simulink model "ReplayAltFilter_oldAtlFilter"  (Simulink 7.8)
settings: Solver=FixedStepDiscrete  StartTime=0.0  StopTime=time(end)  FixedStep=.01  RelTol=1e-3
values from neighbouring files (symbols this model uses):
  apSampleTime = 0.01    [Load_Replay.m]    (also in loadReplayMay2013.m; loadTuneRollReplay_May2013.m; replayFlight.m)
  baroCutoff = 0.2/(2*pi)    (= 0.0318309886184)    [replayFlight.m]
  GS_location = [180 36.9898376464844 -122.051963806152]    [Load_Replay.m]    (also in loadReplayMay2013.m; loadTuneRollReplay_May2013.m; replayFlight.m = [0 36.9898376464844 -122.051963806152])
  ISA_rho0 = 1.225    [replayFlight.m]
  TData = 0.01    [Load_Replay.m]    (also in loadReplayMay2013.m; loadTuneRollReplay_May2013.m)
  Ts = apSampleTime    (= 0.01)    [Load_Replay.m]    (also in loadReplayMay2013.m; loadTuneRollReplay_May2013.m)
  zCutoff = .2    (= 0.2)    [replayFlight.m]
undefined symbols (not defined in the file or in its folder): gaind, polesd, zerosd
libraries: simulink x3
settings Model: Creator=Administrator  LastModifiedBy=Ren
settings OptimizationCC: InitFltsAndDblsToZero=on
settings DebuggingCC: SaveWithParameterizedLinksMsg=none  FcnCallInpInsideContextMsg=Use local settings  StrictBusMsg=Warning
settings SFSimCC: SimParseCustomCode=off
settings GRTTargetCC: TargetFcnLib=ansi_tfl_tmw.mat

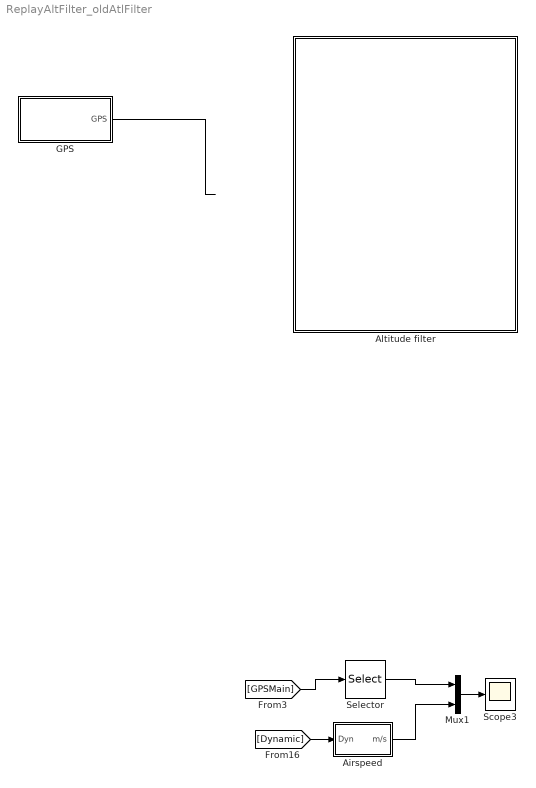
== system ReplayAltFilter_oldAtlFilter ==
  Airspeed : Subsystem
  Altitude filter : Subsystem
  GPS : Subsystem
  Mux1 : Mux  Inputs=2
  Scope3 : Scope
      settings: YMin=0  YMax=22.5  SaveName=ScopeData7
  Selector : Selector  InputPortWidth=5  IndexOptions=Index vector (dialog)  Indices=5  OutputSizes=1
  wires:
  GPS/1(GPS) -> ?
  ? -> ?
  [Dynamic] -> Airspeed/1(Dyn)
  [GPSMain] -> Selector/1
  Selector/1 -> Mux1/1
  Airspeed/1(m/s) -> Mux1/2
  Mux1/1 -> Scope3/1

== system ReplayAltFilter_oldAtlFilter/Airspeed ==
  Dyn : Inport
  Gain : Gain  Gain=2/ISA_rho0
  Math Function : Math  Operator=sqrt  SaturateOnIntegerOverflow=on
  "[0.001  2000]" : Saturate  UpperLimit=2000  LowerLimit=0.001
  m/s : Outport
  wires:
  "[0.001  2000]"/1 -> Math Function/1
  Math Function/1 -> m/s/1
  Dyn/1 -> Gain/1
  Gain/1 -> "[0.001  2000]"/1

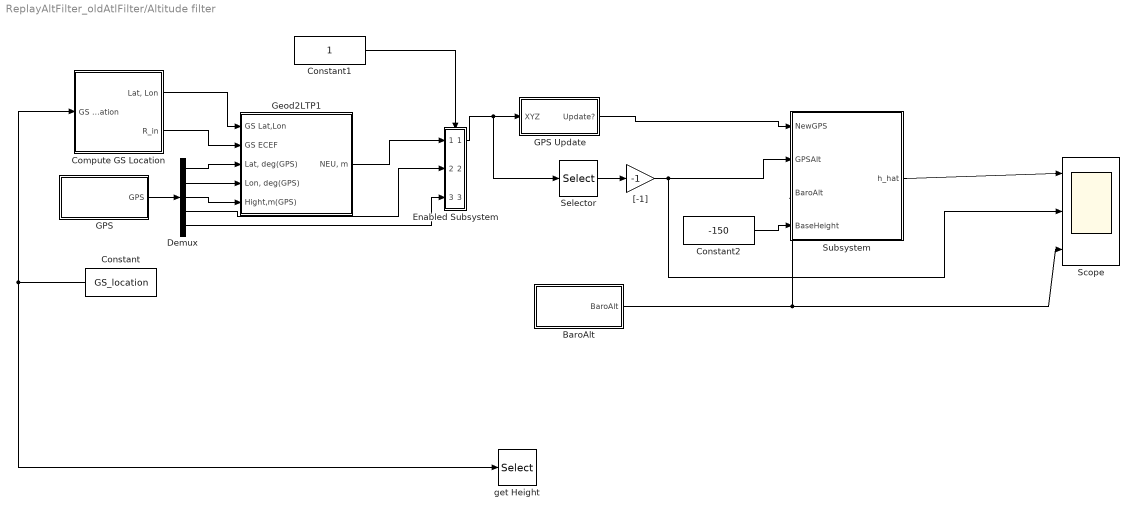
== system ReplayAltFilter_oldAtlFilter/Altitude filter ==
  BaroAlt : Subsystem
  Compute GS Location : Subsystem
  Constant : Constant  Value=GS_location  OutDataTypeStr=single
  Constant1 : Constant  OutDataTypeStr=single
  Constant2 : Constant  Value=-150  OutDataTypeStr=single
  Demux : Demux  Outputs=5
  Enabled Subsystem : Subsystem  TreatAsAtomicUnit=on
  GPS : Subsystem
  GPS Update : Subsystem  mask{T=0.01}
      mask prompts: T "Sample Time"
  Geod2LTP1 : Subsystem
      mask Description:
      | This block provides transformation of the Geodetic coordinates
      | to the LTP coorinate system. The block uses two consecutive transformations
      | (Geodetic -> ECEF ->LTP).
      | Geodetic coordinates of the LTP origin should also be predetermined.
      mask Help: Oops!
      mask Display: plot(0,0,100,100,[45,40,35,40,40],[85,95,85,95,40],[85,95,85,95,40],[35,40,45,40,40],[60,40,10,20,10,14],[70,40,10,13,10,20],[56,45],[70,70],[60,60],[50,60],[60,60],[30,40],[50,60],[20,20],[30,40],[20,20],[45,55],[35,25],[75,65],[35,25])
  Scope : Scope  NumInputPorts=3
      settings: YMin=98550~-50~98550  YMax=99200~15~99300
  Selector : Selector  InputPortWidth=3  IndexOptions=Index vector (dialog)  Indices=[3]  OutputSizes=1
  Subsystem : Subsystem
  "[-1]" : Gain  Gain=-1
  get Height : Selector  InputPortWidth=3  IndexOptions=Index vector (dialog)  Indices=[1]  OutputSizes=1
  wires:
  Constant/1 -> Compute GS Location/1(GS Location), get Height/1
  Demux/1 -> Geod2LTP1/3("Lat, deg(GPS)")
  Demux/2 -> Geod2LTP1/4("Lon, deg(GPS)")
  Demux/3 -> Geod2LTP1/5(Hight,m(GPS))
  Compute GS Location/2(R_in) -> Geod2LTP1/2(GS ECEF)
  Compute GS Location/1("Lat, Lon") -> Geod2LTP1/1(GS Lat,Lon)
  GPS Update/1(Update?) -> Subsystem/1(NewGPS)
  Constant1/1 -> Enabled Subsystem/Enable
  Enabled Subsystem/1(Out1) -> GPS Update/1(XYZ), Selector/1
  Geod2LTP1/1("NEU, m") -> Enabled Subsystem/1(In1)
  Demux/4 -> Enabled Subsystem/2(In2)
  Demux/5 -> Enabled Subsystem/3(In3)
  Subsystem/1(h_hat) -> Scope/1
  Constant2/1 -> Subsystem/4(BaseHeight)
  BaroAlt/1(BaroAlt) -> Subsystem/3(BaroAlt), Scope/3
  "[-1]"/1 -> Subsystem/2(GPSAlt), Scope/2
  Selector/1 -> "[-1]"/1
  GPS/1(GPS) -> Demux/1

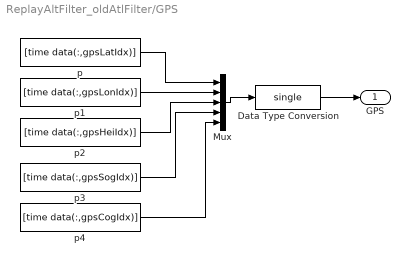
== system ReplayAltFilter_oldAtlFilter/GPS ==
  Data Type Conversion : DataTypeConversion  OutDataTypeStr=single
  Mux : Mux  Inputs=5
  p : FromWorkspace  VariableName=[time data(:,gpsLatIdx)]  SampleTime=TData  OutputAfterFinalValue=Setting to zero
  p1 : FromWorkspace  VariableName=[time data(:,gpsLonIdx)]  SampleTime=TData  OutputAfterFinalValue=Setting to zero
  p2 : FromWorkspace  VariableName=[time data(:,gpsHeiIdx)]  SampleTime=TData  OutputAfterFinalValue=Setting to zero
  p3 : FromWorkspace  VariableName=[time data(:,gpsSogIdx)]  SampleTime=Ts  OutputAfterFinalValue=Setting to zero
  p4 : FromWorkspace  VariableName=[time data(:,gpsCogIdx)]  SampleTime=TData  OutputAfterFinalValue=Setting to zero
  GPS : Outport
  wires:
  p/1 -> Mux/1
  p1/1 -> Mux/2
  p2/1 -> Mux/3
  Mux/1 -> Data Type Conversion/1
  p3/1 -> Mux/4
  p4/1 -> Mux/5
  Data Type Conversion/1 -> GPS/1

== system ReplayAltFilter_oldAtlFilter/Altitude filter/BaroAlt ==
  Data Type Conversion : DataTypeConversion  OutDataTypeStr=single
  p1 : FromWorkspace  VariableName=[time data(:,airStaIdx)]  SampleTime=apSampleTime  OutputAfterFinalValue=Setting to zero
  BaroAlt : Outport
  wires:
  Data Type Conversion/1 -> BaroAlt/1
  p1/1 -> Data Type Conversion/1

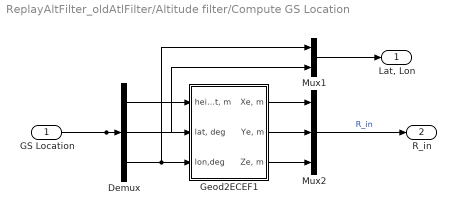
== system ReplayAltFilter_oldAtlFilter/Altitude filter/Compute GS Location ==
  GS Location : Inport
  Demux : Demux  Outputs=3
  Geod2ECEF1 : Subsystem  mask{Re=6378137, Rp=6356752.3142}
      mask prompts: Re "Enter equatorial radius, m"; Rp "Enter polar radius,m"
  Mux1 : Mux  Inputs=2
  Mux2 : Mux  Inputs=3
  "Lat, Lon" : Outport
  R_in : Outport  Port=2
  wires:
  Geod2ECEF1/3("Ze, m ") -> Mux2/3
  Geod2ECEF1/1("Xe, m ") -> Mux2/1
  Geod2ECEF1/2("Ye, m ") -> Mux2/2
  Demux/1 -> Geod2ECEF1/1("height, m")
  Demux/2 -> Mux1/2, Geod2ECEF1/2("lat, deg")
  Demux/3 -> Mux1/1, Geod2ECEF1/3(lon,deg)
  GS Location/1 -> Demux/1
  Mux1/1 -> "Lat, Lon"/1
  Mux2/1 -> R_in/1  "R_in"

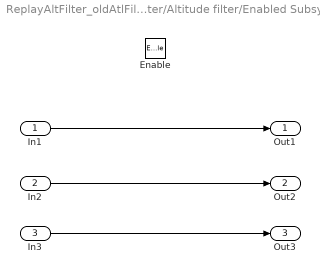
== system ReplayAltFilter_oldAtlFilter/Altitude filter/Enabled Subsystem ==
  In1 : Inport
  In2 : Inport  Port=2
  In3 : Inport  Port=3
  Enable : EnablePort
  Out1 : Outport
  Out2 : Outport  Port=2
  Out3 : Outport  Port=3
  wires:
  In1/1 -> Out1/1
  In2/1 -> Out2/1
  In3/1 -> Out3/1

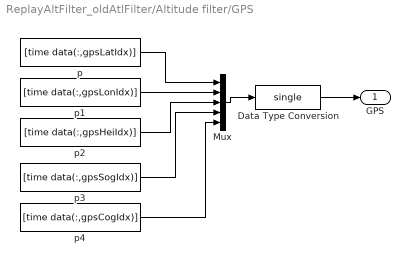
== system ReplayAltFilter_oldAtlFilter/Altitude filter/GPS ==
  Data Type Conversion : DataTypeConversion  OutDataTypeStr=single
  Mux : Mux  Inputs=5
  p : FromWorkspace  VariableName=[time data(:,gpsLatIdx)]  SampleTime=TData  OutputAfterFinalValue=Setting to zero
  p1 : FromWorkspace  VariableName=[time data(:,gpsLonIdx)]  SampleTime=TData  OutputAfterFinalValue=Setting to zero
  p2 : FromWorkspace  VariableName=[time data(:,gpsHeiIdx)]  SampleTime=TData  OutputAfterFinalValue=Setting to zero
  p3 : FromWorkspace  VariableName=[time data(:,gpsSogIdx)]  SampleTime=Ts  OutputAfterFinalValue=Setting to zero
  p4 : FromWorkspace  VariableName=[time data(:,gpsCogIdx)]  SampleTime=TData  OutputAfterFinalValue=Setting to zero
  GPS : Outport
  wires:
  p/1 -> Mux/1
  p1/1 -> Mux/2
  p2/1 -> Mux/3
  Mux/1 -> Data Type Conversion/1
  p3/1 -> Mux/4
  p4/1 -> Mux/5
  Data Type Conversion/1 -> GPS/1

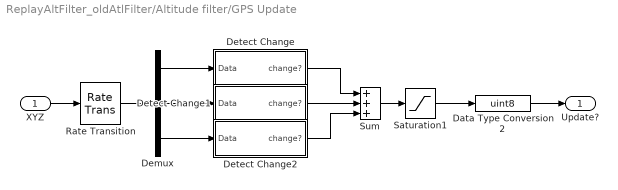
== system ReplayAltFilter_oldAtlFilter/Altitude filter/GPS Update ==
  XYZ : Inport
  Data Type Conversion2 : DataTypeConversion  OutDataTypeStr=uint8
  Demux : Demux  Outputs=3
  Detect Change : Subsystem
  Detect Change1 : Subsystem
  Detect Change2 : Subsystem
  Rate Transition : RateTransition  OutPortSampleTime=T
  Saturation1 : Saturate  UpperLimit=1  LowerLimit=0  SampleTime=T
  Sum : Sum  Inputs=3
  Update? : Outport
  wires:
  Demux/1 -> Detect Change/1(Data)
  Demux/2 -> Detect Change1/1(Data)
  Demux/3 -> Detect Change2/1(Data)
  Detect Change/1(change?) -> Sum/1
  Detect Change1/1(change?) -> Sum/2
  Detect Change2/1(change?) -> Sum/3
  Sum/1 -> Saturation1/1
  XYZ/1 -> Rate Transition/1
  Saturation1/1 -> Data Type Conversion2/1
  Rate Transition/1 -> Demux/1
  Data Type Conversion2/1 -> Update?/1

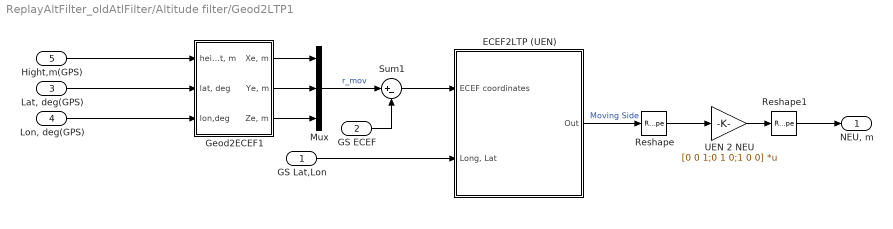
== system ReplayAltFilter_oldAtlFilter/Altitude filter/Geod2LTP1 ==
  GS Lat,Lon : Inport
  GS ECEF : Inport  Port=2
  "Lat, deg(GPS)" : Inport  Port=3
  "Lon, deg(GPS)" : Inport  Port=4
  Hight,m(GPS) : Inport  Port=5
  ECEF2LTP (UEN) : Subsystem
      mask Display: plot(0,0,100,100,[45,40,35,40,40],[85,95,85,95,40],[85,95,85,95,40],[35,40,45,40,40],[60,40,10,20,10,14],[70,40,10,13,10,20],[56,45],[70,70],[60,60],[50,60],[60,60],[30,40],[50,60],[20,20],[30,40],[20,20],[45,55],[35,25],[75,65],[35,25])
  Geod2ECEF1 : Subsystem  mask{Re=6378137, Rp=6356752.3142}
      mask prompts: Re "Enter equatorial radius, m"; Rp "Enter polar radius,m"
  Mux : Mux  Inputs=3
  Reshape : Reshape  OutputDimensionality=Column vector (2-D)
  Reshape1 : Reshape
  Sum1 : Sum  Inputs=|+-  OutDataTypeStr=single  SaturateOnIntegerOverflow=on
  UEN 2 NEU : Gain  Gain=[0 0 1;0 1 0;1 0 0]  Multiplication=Matrix(K*u)  OutDataTypeStr=float('single')  SaturateOnIntegerOverflow=on  ParamDataTypeStr=Inherit: Same as input
  "NEU, m" : Outport
  wires:
  Reshape1/1 -> "NEU, m"/1
  Reshape/1 -> UEN 2 NEU/1
  Sum1/1 -> ECEF2LTP (UEN)/1(ECEF coordinates)
  Mux/1 -> Sum1/1  "r_mov"
  Hight,m(GPS)/1 -> Geod2ECEF1/1("height, m")
  ECEF2LTP (UEN)/1(Out) -> Reshape/1  "Moving Side"
  GS ECEF/1 -> Sum1/2
  GS Lat,Lon/1 -> ECEF2LTP (UEN)/2("Long, Lat")
  "Lon, deg(GPS)"/1 -> Geod2ECEF1/3(lon,deg)
  "Lat, deg(GPS)"/1 -> Geod2ECEF1/2("lat, deg")
  Geod2ECEF1/2("Ye, m ") -> Mux/2
  Geod2ECEF1/1("Xe, m ") -> Mux/1
  Geod2ECEF1/3("Ze, m ") -> Mux/3
  UEN 2 NEU/1 -> Reshape1/1

== system ReplayAltFilter_oldAtlFilter/Altitude filter/Subsystem ==
  NewGPS : Inport
  GPSAlt : Inport  Port=2
  BaroAlt : Inport  Port=3
  BaseHeight : Inport  Port=4
  2 FIlter Blend : Subsystem
  h_hat : Outport
  wires:
  2 FIlter Blend/1(Blend) -> h_hat/1
  BaseHeight/1 -> 2 FIlter Blend/4(baseHeight)
  BaroAlt/1 -> 2 FIlter Blend/2(BaroAlt)
  GPSAlt/1 -> 2 FIlter Blend/1(gps_h)
  NewGPS/1 -> 2 FIlter Blend/3(New GPS)

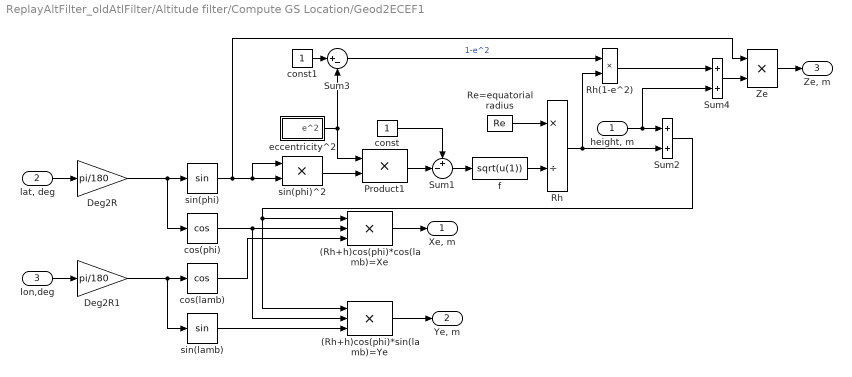
== system ReplayAltFilter_oldAtlFilter/Altitude filter/Compute GS Location/Geod2ECEF1 ==
  "height, m" : Inport
  "lat, deg" : Inport  Port=2
  lon,deg : Inport  Port=3
  (Rh+h)cos(phi)*cos(lamb)=Xe : Product  Inputs=3  OutDataTypeStr=single  SaturateOnIntegerOverflow=on  InputSameDT=on
  (Rh+h)cos(phi)*sin(lamb)=Ye : Product  Inputs=3  OutDataTypeStr=single  SaturateOnIntegerOverflow=on  InputSameDT=on
  Deg2R : Gain  Gain=pi/180  OutDataTypeStr=float('single')  SaturateOnIntegerOverflow=on  ParamDataTypeStr=Inherit: Same as input
  Deg2R1 : Gain  Gain=pi/180  OutDataTypeStr=float('single')  SaturateOnIntegerOverflow=on  ParamDataTypeStr=Inherit: Same as input
  Product1 : Product  SaturateOnIntegerOverflow=on  InputSameDT=on  OutDataTypeStr=Inherit: Same as first input
  Re=equatorial radius : Constant  Value=Re  OutDataTypeStr=single
  Rh : Product  Inputs=*/  OutDataTypeStr=single  SaturateOnIntegerOverflow=on  InputSameDT=on
  Rh(1-e^2) : Product  OutDataTypeStr=single  SaturateOnIntegerOverflow=on  InputSameDT=on
  Sum1 : Sum  Inputs=+-|  SaturateOnIntegerOverflow=on  InputSameDT=on  OutDataTypeStr=Inherit: Same as first input
  Sum2 : Sum  SaturateOnIntegerOverflow=on  InputSameDT=on  OutDataTypeStr=Inherit: Same as first input
      settings: AttributesFormatString=Rh+h
  Sum3 : Sum  Inputs=|+-  SaturateOnIntegerOverflow=on  InputSameDT=on  OutDataTypeStr=Inherit: Same as first input
  Sum4 : Sum  OutDataTypeStr=single  SaturateOnIntegerOverflow=on  InputSameDT=on
      settings: AttributesFormatString=(1-e^2)Rh+h
  Ze : Product  OutDataTypeStr=single  SaturateOnIntegerOverflow=on  InputSameDT=on
  const : Constant  OutDataTypeStr=single
  const1 : Constant  OutDataTypeStr=single
  cos(lamb) : Trigonometry  Operator=cos
  cos(phi) : Trigonometry  Operator=cos
  eccentricity^2 : Subsystem
  f : Fcn  Expr=sqrt(u(1))
  sin(lamb) : Trigonometry
  sin(phi) : Trigonometry
  sin(phi)^2 : Product  SaturateOnIntegerOverflow=on  InputSameDT=on  OutDataTypeStr=Inherit: Same as first input
  "Xe, m " : Outport
  "Ye, m " : Outport  Port=2
  "Ze, m " : Outport  Port=3
  wires:
  (Rh+h)cos(phi)*sin(lamb)=Ye/1 -> "Ye, m "/1
  (Rh+h)cos(phi)*cos(lamb)=Xe/1 -> "Xe, m "/1
  Sum2/1 -> (Rh+h)cos(phi)*cos(lamb)=Xe/1, (Rh+h)cos(phi)*sin(lamb)=Ye/1
  Deg2R1/1 -> sin(lamb)/1, cos(lamb)/1
  Deg2R/1 -> sin(phi)/1, cos(phi)/1
  Ze/1 -> "Ze, m "/1
  sin(lamb)/1 -> (Rh+h)cos(phi)*sin(lamb)=Ye/3
  cos(lamb)/1 -> (Rh+h)cos(phi)*cos(lamb)=Xe/3
  cos(phi)/1 -> (Rh+h)cos(phi)*sin(lamb)=Ye/2, (Rh+h)cos(phi)*cos(lamb)=Xe/2
  lon,deg/1 -> Deg2R1/1
  Sum4/1 -> Ze/2
  Rh(1-e^2)/1 -> Sum4/1
  Sum3/1 -> Rh(1-e^2)/1  "1-e^2"
  const1/1 -> Sum3/1
  sin(phi)^2/1 -> Product1/2
  eccentricity^2/1(e^2) -> Sum3/2, Product1/1
  "height, m"/1 -> Sum2/1, Sum4/2
  const/1 -> Sum1/1
  Sum1/1 -> f/1
  Product1/1 -> Sum1/2
  Rh/1 -> Rh(1-e^2)/2, Sum2/2
  Re=equatorial radius/1 -> Rh/1
  f/1 -> Rh/2
  sin(phi)/1 -> Ze/1, sin(phi)^2/2, sin(phi)^2/1
  "lat, deg"/1 -> Deg2R/1

== system ReplayAltFilter_oldAtlFilter/Altitude filter/GPS Update/Detect Change ==
  Data : Inport
  Abs1 : Abs  SampleTime=T
  Difference1 : simulink/Discrete/Difference  ICPrevInput=0.0  InputProcessing=Inherited  OutMin=[]  OutMax=[]  OutDataType=sfix(16)  OutScaling=2^-10  DoSatur=off
  Saturation1 : Saturate  UpperLimit=1  LowerLimit=0  SampleTime=T
  change? : Outport
  wires:
  Difference1/1 -> Abs1/1
  Abs1/1 -> Saturation1/1
  Data/1 -> Difference1/1
  Saturation1/1 -> change?/1

== system ReplayAltFilter_oldAtlFilter/Altitude filter/GPS Update/Detect Change1 ==
  Data : Inport
  Abs1 : Abs  SampleTime=T
  Difference1 : simulink/Discrete/Difference  ICPrevInput=0.0  InputProcessing=Inherited  OutMin=[]  OutMax=[]  OutDataType=sfix(16)  OutScaling=2^-10  DoSatur=off
  Saturation1 : Saturate  UpperLimit=1  LowerLimit=0  SampleTime=T
  change? : Outport
  wires:
  Saturation1/1 -> change?/1
  Data/1 -> Difference1/1
  Abs1/1 -> Saturation1/1
  Difference1/1 -> Abs1/1

== system ReplayAltFilter_oldAtlFilter/Altitude filter/GPS Update/Detect Change2 ==
  Data : Inport
  Abs1 : Abs  SampleTime=T
  Difference1 : simulink/Discrete/Difference  ICPrevInput=0.0  InputProcessing=Inherited  OutMin=[]  OutMax=[]  OutDataType=sfix(16)  OutScaling=2^-10  DoSatur=off
  Saturation1 : Saturate  UpperLimit=1  LowerLimit=0  SampleTime=T
  change? : Outport
  wires:
  Difference1/1 -> Abs1/1
  Abs1/1 -> Saturation1/1
  Data/1 -> Difference1/1
  Saturation1/1 -> change?/1

== system ReplayAltFilter_oldAtlFilter/Altitude filter/Geod2LTP1/ECEF2LTP (UEN) ==
  ECEF coordinates : Inport
  "Long, Lat" : Inport  Port=2
  Deg2R : Gain  Gain=pi/180  SaturateOnIntegerOverflow=on  OutDataTypeStr=Inherit: Same as input  ParamDataTypeStr=Inherit: Same as input
  Demux3 : Demux  Outputs=2
  From Body to Universal1 : Subsystem
  Product1 : Product  Multiplication=Matrix(*)  SaturateOnIntegerOverflow=on  InputSameDT=on  OutDataTypeStr=Inherit: Same as first input
  Out : Outport
  wires:
  From Body to Universal1/1(DCM) -> Product1/1
  ECEF coordinates/1 -> Product1/2
  Deg2R/1 -> Demux3/1
  Demux3/1 -> From Body to Universal1/1(long)
  Demux3/2 -> From Body to Universal1/2(lat)
  Product1/1 -> Out/1
  "Long, Lat"/1 -> Deg2R/1

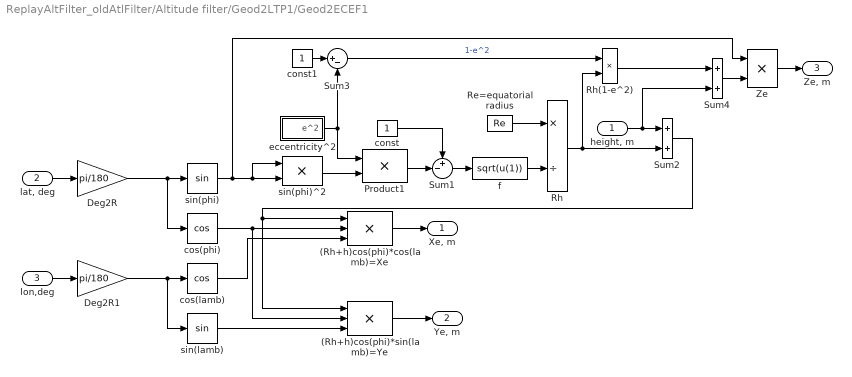
== system ReplayAltFilter_oldAtlFilter/Altitude filter/Geod2LTP1/Geod2ECEF1 ==
  "height, m" : Inport
  "lat, deg" : Inport  Port=2
  lon,deg : Inport  Port=3
  (Rh+h)cos(phi)*cos(lamb)=Xe : Product  Inputs=3  OutDataTypeStr=single  SaturateOnIntegerOverflow=on  InputSameDT=on
  (Rh+h)cos(phi)*sin(lamb)=Ye : Product  Inputs=3  OutDataTypeStr=single  SaturateOnIntegerOverflow=on  InputSameDT=on
  Deg2R : Gain  Gain=pi/180  OutDataTypeStr=float('single')  SaturateOnIntegerOverflow=on  ParamDataTypeStr=Inherit: Same as input
  Deg2R1 : Gain  Gain=pi/180  OutDataTypeStr=float('single')  SaturateOnIntegerOverflow=on  ParamDataTypeStr=Inherit: Same as input
  Product1 : Product  SaturateOnIntegerOverflow=on  InputSameDT=on  OutDataTypeStr=Inherit: Same as first input
  Re=equatorial radius : Constant  Value=Re  OutDataTypeStr=single
  Rh : Product  Inputs=*/  OutDataTypeStr=single  SaturateOnIntegerOverflow=on  InputSameDT=on
  Rh(1-e^2) : Product  OutDataTypeStr=single  SaturateOnIntegerOverflow=on  InputSameDT=on
  Sum1 : Sum  Inputs=+-|  SaturateOnIntegerOverflow=on  InputSameDT=on  OutDataTypeStr=Inherit: Same as first input
  Sum2 : Sum  SaturateOnIntegerOverflow=on  InputSameDT=on  OutDataTypeStr=Inherit: Same as first input
      settings: AttributesFormatString=Rh+h
  Sum3 : Sum  Inputs=|+-  SaturateOnIntegerOverflow=on  InputSameDT=on  OutDataTypeStr=Inherit: Same as first input
  Sum4 : Sum  OutDataTypeStr=single  SaturateOnIntegerOverflow=on  InputSameDT=on
      settings: AttributesFormatString=(1-e^2)Rh+h
  Ze : Product  OutDataTypeStr=single  SaturateOnIntegerOverflow=on  InputSameDT=on
  const : Constant  OutDataTypeStr=single
  const1 : Constant  OutDataTypeStr=single
  cos(lamb) : Trigonometry  Operator=cos
  cos(phi) : Trigonometry  Operator=cos
  eccentricity^2 : Subsystem
  f : Fcn  Expr=sqrt(u(1))
  sin(lamb) : Trigonometry
  sin(phi) : Trigonometry
  sin(phi)^2 : Product  SaturateOnIntegerOverflow=on  InputSameDT=on  OutDataTypeStr=Inherit: Same as first input
  "Xe, m " : Outport
  "Ye, m " : Outport  Port=2
  "Ze, m " : Outport  Port=3
  wires:
  (Rh+h)cos(phi)*sin(lamb)=Ye/1 -> "Ye, m "/1
  (Rh+h)cos(phi)*cos(lamb)=Xe/1 -> "Xe, m "/1
  Sum2/1 -> (Rh+h)cos(phi)*cos(lamb)=Xe/1, (Rh+h)cos(phi)*sin(lamb)=Ye/1
  Deg2R1/1 -> sin(lamb)/1, cos(lamb)/1
  Deg2R/1 -> sin(phi)/1, cos(phi)/1
  Ze/1 -> "Ze, m "/1
  sin(lamb)/1 -> (Rh+h)cos(phi)*sin(lamb)=Ye/3
  cos(lamb)/1 -> (Rh+h)cos(phi)*cos(lamb)=Xe/3
  cos(phi)/1 -> (Rh+h)cos(phi)*sin(lamb)=Ye/2, (Rh+h)cos(phi)*cos(lamb)=Xe/2
  lon,deg/1 -> Deg2R1/1
  Sum4/1 -> Ze/2
  Rh(1-e^2)/1 -> Sum4/1
  Sum3/1 -> Rh(1-e^2)/1  "1-e^2"
  const1/1 -> Sum3/1
  sin(phi)^2/1 -> Product1/2
  eccentricity^2/1(e^2) -> Sum3/2, Product1/1
  "height, m"/1 -> Sum2/1, Sum4/2
  const/1 -> Sum1/1
  Sum1/1 -> f/1
  Product1/1 -> Sum1/2
  Rh/1 -> Rh(1-e^2)/2, Sum2/2
  Re=equatorial radius/1 -> Rh/1
  f/1 -> Rh/2
  sin(phi)/1 -> Ze/1, sin(phi)^2/2, sin(phi)^2/1
  "lat, deg"/1 -> Deg2R/1

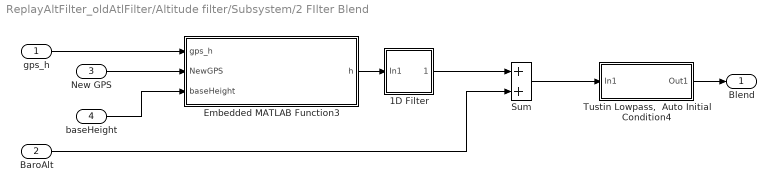
== system ReplayAltFilter_oldAtlFilter/Altitude filter/Subsystem/2 FIlter Blend ==
  gps_h : Inport
  BaroAlt : Inport  Port=2
  New GPS : Inport  Port=3
  baseHeight : Inport  Port=4
  1D Filter : Subsystem  AncestorBlock=SLUGS_Library/Singnal Routing & Conditioning/3D Filter  RTWFcnName=TustinFilter3D  mask{zval=[0], pval=-zCutoff, kval=1, TSample=apSampleTime}
      mask prompts: zval "Zeros"; pval "Poles"; kval "Gains"; TSample "Sample Time"
      settings: RTWFcnNameOpts=User specified  RTWFileNameOpts=Use function name
      mask Display:
      | droots(zval,pval,kval)
      | port_label('input',1,'1D')
  Embedded MATLAB Function3 : MATLAB Function  TreatAsAtomicUnit=on
  Sum : Sum  OutDataTypeStr=single
  "Tustin Lowpass,  Auto Initial Condition4" : Subsystem  mask(Tustin1stOrderLowpassAutoInitialCondition){f=baroCutoff, T=apSampleTime}
      mask prompts: f "Lowpass Frequency"; T "Sample Time"
      mask help: Takes a 3db rolloff frequency (in Hz, NOT radians/s) and a sample time. Performs a symbolic Tustin conversion and implements in a discrete filter. The initial output of the filter is set by the first sample.
      mask Help: Enter the desired 3db rolloff frequency in Hz and the sample time. Initial conditions are sampled automatically.
      mask Display: fprintf('%.2f Hz lowpass',f)
  Blend : Outport
  wires:
  BaroAlt/1 -> Sum/2
  1D Filter/1(Out1) -> Sum/1
  Sum/1 -> "Tustin Lowpass,  Auto Initial Condition4"/1(In1)
  New GPS/1 -> Embedded MATLAB Function3/2(NewGPS)
  gps_h/1 -> Embedded MATLAB Function3/1(gps_h)
  Embedded MATLAB Function3/1(h) -> 1D Filter/1(In1)
  baseHeight/1 -> Embedded MATLAB Function3/3(baseHeight)
  "Tustin Lowpass,  Auto Initial Condition4"/1(Out1) -> Blend/1

== system ReplayAltFilter_oldAtlFilter/Altitude filter/Compute GS Location/Geod2ECEF1/eccentricity^2 ==
  " " : Product  OutDataTypeStr=single  SaturateOnIntegerOverflow=on  InputSameDT=on
  Re=equatorial radius1 : Constant  Value=Re  OutDataTypeStr=single
  Rp=polar radius : Constant  Value=Rp  OutDataTypeStr=single
  Sum5 : Sum  Inputs=|+-  SaturateOnIntegerOverflow=on  InputSameDT=on  OutDataTypeStr=Inherit: Same as first input
  const2 : Constant  OutDataTypeStr=single
  e^1 : Product  Inputs=*/  OutDataTypeStr=single  SaturateOnIntegerOverflow=on  InputSameDT=on
  e^2 : Outport
  wires:
  Sum5/1 -> e^2/1
  " "/1 -> Sum5/2
  e^1/1 -> " "/1, " "/2
  const2/1 -> Sum5/1
  Rp=polar radius/1 -> e^1/1
  Re=equatorial radius1/1 -> e^1/2

== system ReplayAltFilter_oldAtlFilter/Altitude filter/Geod2LTP1/ECEF2LTP (UEN)/From Body to Universal1 ==
  long : Inport
  lat : Inport  Port=2
  Mux : Mux  Inputs=2
  Reshape 9x1->3x1 : Reshape  OutputDimensionality=Customize  OutputDimensions=[3,3]
  Rotation Matrix from Long//Lat : Subsystem
      mask Type: Vector Transformation
      mask Description: Vector Transformation
      mask Display: disp('axis')
  DCM : Outport
  wires:
  Reshape 9x1->3x1/1 -> DCM/1
  Rotation Matrix from Long//Lat/1(DCM) -> Reshape 9x1->3x1/1
  Mux/1 -> Rotation Matrix from Long//Lat/1(long lat)
  long/1 -> Mux/1
  lat/1 -> Mux/2

== system ReplayAltFilter_oldAtlFilter/Altitude filter/Geod2LTP1/Geod2ECEF1/eccentricity^2 ==
  " " : Product  OutDataTypeStr=single  SaturateOnIntegerOverflow=on  InputSameDT=on
  Re=equatorial radius1 : Constant  Value=Re  OutDataTypeStr=single
  Rp=polar radius : Constant  Value=Rp  OutDataTypeStr=single
  Sum5 : Sum  Inputs=|+-  SaturateOnIntegerOverflow=on  InputSameDT=on  OutDataTypeStr=Inherit: Same as first input
  const2 : Constant  OutDataTypeStr=single
  e^1 : Product  Inputs=*/  OutDataTypeStr=single  SaturateOnIntegerOverflow=on  InputSameDT=on
  e^2 : Outport
  wires:
  Sum5/1 -> e^2/1
  " "/1 -> Sum5/2
  e^1/1 -> " "/1, " "/2
  const2/1 -> Sum5/1
  Rp=polar radius/1 -> e^1/1
  Re=equatorial radius1/1 -> e^1/2

== system ReplayAltFilter_oldAtlFilter/Altitude filter/Subsystem/2 FIlter Blend/1D Filter ==
  In1 : Inport
  Data Type Conversion1 : DataTypeConversion  OutDataTypeStr=single
  Data Type Conversion2 : DataTypeConversion  OutDataTypeStr=double
  Filter2 : Subsystem  mask(DiscretizedZeroPole){Zeros=zval, Poles=pval, Gain=kval, AbsTol=auto, SampleTime=TSample, method=tustin, Wc=1}
      mask prompts: Zeros "Zeros (enter in s-main:)"; Poles "Poles (enter in s-domain:)"; Gain "Gain (enter in s-domain:)"; AbsTol "Absolute tolerance:"; SampleTime "Sample time:"; Wc "Critical Frequency (Hz):"
      mask help: Continuous mask uses c2d to transform parameters onto the Discrete Zero-Pole block inside.
      mask init:
      | st=SampleTime;
      | if length(st)>1
      |     st=SampleTime(1);
      | end
      | if(st>0)
      |     [zerosd,polesd,gaind] = sldiscutil('disczpk', {st,method,Wc,Zeros,Poles,Gain});
      | end	
      | s = get_param(gcb,'maskvalues');
      | zeross = s{1};
      | poless = s{2};
      | gainss = s{3};
      | %zerosc = eval(zeross);
      | %polesc = eval(poless);
      | %gainsc = eval(gainss);
      | sldiscutil('initzpkmask', st);
      | if(st==0)
      | set_param([gcb '/Zero Pole'], 'AbsoluteTolerance', AbsTol);
      | end
      mask StyleString: edit,edit,edit,edit,edit,popup(zoh|foh|tustin|prewarp|matched),edit
      mask CallbackString: |||||hidecrit|
      mask Display:
      | droots(zeross,poless,gainss)
      | text( 0.5, 1.0, method, 'verticalAlignment','top')
  Out1 : Outport
  wires:
  Data Type Conversion1/1 -> Out1/1
  Data Type Conversion2/1 -> Filter2/1(In1)
  In1/1 -> Data Type Conversion2/1
  Filter2/1(Out1) -> Data Type Conversion1/1

== system ReplayAltFilter_oldAtlFilter/Altitude filter/Subsystem/2 FIlter Blend/Tustin Lowpass,  Auto Initial Condition4 ==
  In1 : Inport
  Constant : Constant  Value=T
  Constant1 : Constant  Value=f
  Embedded MATLAB Function : MATLAB Function  TreatAsAtomicUnit=on
  Out1 : Outport
  wires:
  Constant/1 -> Embedded MATLAB Function/2(T)
  Constant1/1 -> Embedded MATLAB Function/3(f)
  Embedded MATLAB Function/1(y) -> Out1/1
  In1/1 -> Embedded MATLAB Function/1(u)

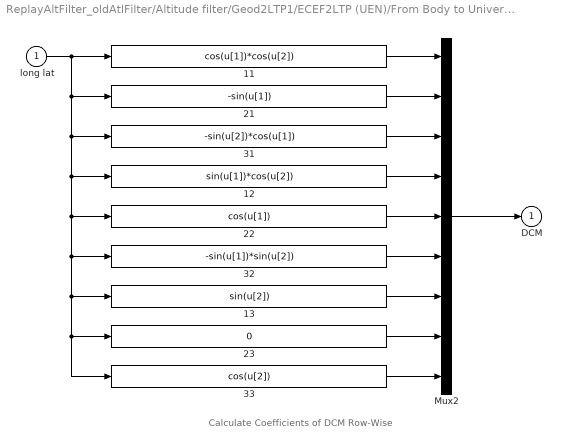
== system ReplayAltFilter_oldAtlFilter/Altitude filter/Geod2LTP1/ECEF2LTP (UEN)/From Body to Universal1/Rotation Matrix from Long//Lat ==
  note: Calculate Coefficients of DCM Row-Wise
  long lat : Inport
  11 : Fcn  Expr=cos(u[1])*cos(u[2])
  12 : Fcn  Expr=sin(u[1])*cos(u[2])
  13 : Fcn  Expr=sin(u[2])
  21 : Fcn  Expr=-sin(u[1])
  22 : Fcn  Expr=cos(u[1])
  23 : Fcn  Expr=0
  31 : Fcn  Expr=-sin(u[2])*cos(u[1])
  32 : Fcn  Expr=-sin(u[1])*sin(u[2])
  33 : Fcn  Expr=cos(u[2])
  Mux2 : Mux  Inputs=9
  DCM : Outport
  wires:
  long lat/1 -> 21/1, 31/1, 12/1, 22/1, 32/1, 13/1, 23/1, 33/1, 11/1
  Mux2/1 -> DCM/1
  11/1 -> Mux2/1
  21/1 -> Mux2/2
  31/1 -> Mux2/3
  12/1 -> Mux2/4
  22/1 -> Mux2/5
  32/1 -> Mux2/6
  13/1 -> Mux2/7
  23/1 -> Mux2/8
  33/1 -> Mux2/9

== system ReplayAltFilter_oldAtlFilter/Altitude filter/Subsystem/2 FIlter Blend/1D Filter/Filter2 ==
  In1 : Inport
  Discrete Zero-Pole : DiscreteZeroPole  Zeros=zerosd  Poles=polesd  Gain=gaind  SampleTime=SampleTime
  Out1 : Outport
  wires:
  Discrete Zero-Pole/1 -> Out1/1
  In1/1 -> Discrete Zero-Pole/1

== matlab function Altitude filter/Subsystem/2 FIlter Blend/Tustin Lowpass, Auto Initial Condition4/Embedded MATLAB Function ==
  data: u input double; y output double; T input double; f input double
function y = fcn(u,T,f)
% This block supports an embeddable subset of the MATLAB language.
% See the help menu for details. 

persistent a
persistent b
persistent y_km1
persistent u_km1
if isempty(a)
    %tf = [T*omega/(2+T*omega) T*omega/(2+T*omega)],[1 (T*omega-2)/(T*omega+2)]
    %tf = [a a],[1 -b]
    omega = 2*pi*f;
    a=T*omega/(2+T*omega);
    b=-(T*omega-2)/(T*omega+2);
    y_km1=u;
    u_km1=u;
end

y = a*(u+u_km1)+b*y_km1;
y_km1=y;
u_km1=u;

== matlab function Altitude filter/Subsystem/2 FIlter Blend/Embedded MATLAB Function3 ==
  data: gps_h input double size=1; h output double size=1; NewGPS input double size=1; apSampleTime parameter double size=1; baseHeight input double
function h = heightRateAid(gps_h,NewGPS,apSampleTime, baseHeight)
persistent lastGps_h;
persistent TimeSinceLast;
persistent rate;
persistent lastH;

if (isempty(lastGps_h))
    lastGps_h       = single(0.0);
    TimeSinceLast   = single(apSampleTime);
    rate            = single(0);
    lastH           = single(-baseHeight);
end

if (NewGPS)
    rate = single((gps_h - lastGps_h)/TimeSinceLast);
    TimeSinceLast = single(0);
    if (rate > -10.6) && (rate < 17.67)
        h = lastH + gps_h - lastGps_h;
    else
        h = lastH;
    end
    lastGps_h = gps_h;
else
    h = lastH;
end

TimeSinceLast = TimeSinceLast + apSampleTime;
lastH = h;
